simulink model "sl_rrmc"  (R2015a)
settings: Solver=ode45  StartTime=0.0  StopTime=5.0  RelTol=1e-3
undefined symbols (not defined in the file): DiscIntNeverNeededParam
libraries: roblocks x2
settings Model: ExtModeAutoUpdateStatusClock=off  Creator=pic  LastModifiedBy=corkep
settings DataIOCC: LimitDataPoints=off  SignalLoggingSaveFormat=ModelDataLogs  ReturnWorkspaceOutputs=on  SignalLoggingName=sigsOut
settings OptimizationCC: ExpressionDepthLimit=2147483647
settings DebuggingCC: SaveWithParameterizedLinksMsg=none  UnderspecifiedInitializationDetection=Classic  MergeDetectMultiDrivingBlocksExec=none  SignalResolutionControl=TryResolveAllWithWarning  MultiTaskDSMMsg=warning  MultiTaskCondExecSysMsg=none  FcnCallInpInsideContextMsg=EnableAllAsWarning  StateNameClashWarn=warning
settings HardwareCC: TargetUnknown=on
settings GRTTargetCC: CombineOutputUpdateFcns=off  GRTInterface=on

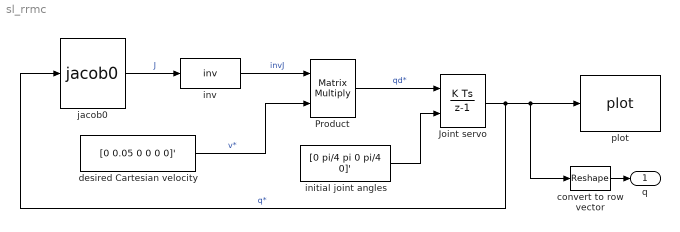
== system sl_rrmc ==
  Joint servo : DiscreteIntegrator  InitialConditionSource=external  InitialCondition=[0 pi/4 pi 0 pi/4 0]'  InitialConditionSetting=State (most efficient)  SampleTime=0.05  ICPrevOutput=DiscIntNeverNeededParam  ICPrevScaledInput=DiscIntNeverNeededParam
  Product : Product  Multiplication=Matrix(*)  SaturateOnIntegerOverflow=on  OutDataTypeStr=Inherit: Same as first input
  convert to row vector : Reshape  OutputDimensionality=Customize  OutputDimensions=6
  desired Cartesian velocity : Constant  Value=[0 0.05 0 0 0 0]'  VectorParams1D=off
  initial joint angles : Constant  Value="[0 pi/4 pi  0 pi/4 0]'"  VectorParams1D=off
  inv : MATLABFcn  MATLABFcn=inv  Output1D=off
  "jacob0 " : roblocks/Arm/jacob0   robot=p560
  plot : roblocks/Arm/plot  robot=p560  fps=25  holdplot=on
  q : Outport
  wires:
  "jacob0 "/1 -> inv/1  "J"
  Joint servo/1 -> plot/1, convert to row vector/1, "jacob0 "/1  "q*"
  inv/1 -> Product/1  "invJ"
  desired Cartesian velocity/1 -> Product/2  "v*"
  convert to row vector/1 -> q/1
  Product/1 -> Joint servo/1  "qd*"
  initial joint angles/1 -> Joint servo/2
